simulink model "nonlinear_gate"  (R2025b)
settings: Solver=VariableStepAuto  StartTime=0.0  StopTime=10.0  FixedStep=1e-5  RelTol=1e-3
settings Model: Creator=LYG  LastModifiedBy=LYG

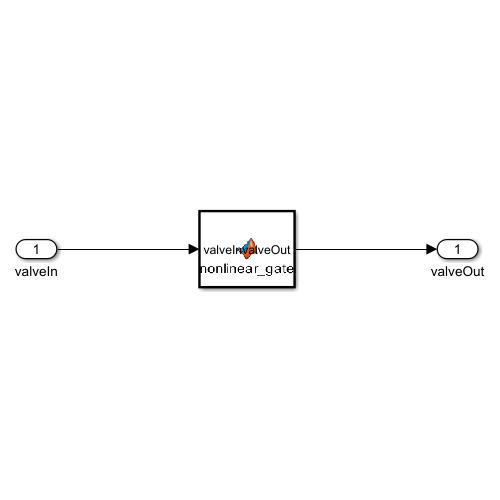
[thumbnail: Simulink's stored preview of the top-level diagram]
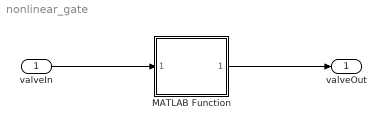
== system nonlinear_gate ==
  valveIn : Inport
  MATLAB Function : MATLAB Function  TreatAsAtomicUnit=on
  valveOut : Outport
  wires:
  valveIn/1 -> MATLAB Function/1(valveIn)
  MATLAB Function/1(valveOut) -> valveOut/1

== matlab function nonlinear_gate/MATLAB Function ==
  data: valveIn input; valveOut output
function valveOut = nonlinear_gate(valveIn)
    % Parameters
    eps = 1e-3;
    dl = -0.014; dr = 0.014;
    kl = 0.0276; kr = 0.04;
    Sl = -0.004; Sr = 0.006;
    
    % voltage-speed characteristic
    valveOut = zeros(1);
    softplus_l = eps * log(1 + exp((dl - valveIn) / eps));
    softplus_r = eps * log(1 + exp((valveIn - dr) / eps));
    w_soft = kr * softplus_r - kl * softplus_l;
    if valveIn >= 0
        valveOut(1) = Sr * tanh(w_soft / Sr);
    else
        valveOut(1) = Sl * tanh(w_soft / Sl);
    end
end
